simulink model "iasted_s1"  (R2014a)
settings: Solver=ode3  StartTime=0.0  StopTime=10  FixedStep=T  RelTol=1e-3
values from neighbouring files (symbols this model uses):
  amplitude = 10    [iasted_m1.m]
  duracao = 0.1    [iasted_m1.m]
  G = [solution.k1  solution.k2  0  solution.k4]    [iasted_m1.m]
  theta_r = 1.0    (= 1)    [iasted_m1.m]
  ti = 10    [iasted_m1.m]
settings Model: Creator=fabrizio  LastModifiedBy=fabrizio
settings DataIOCC: Refine=10

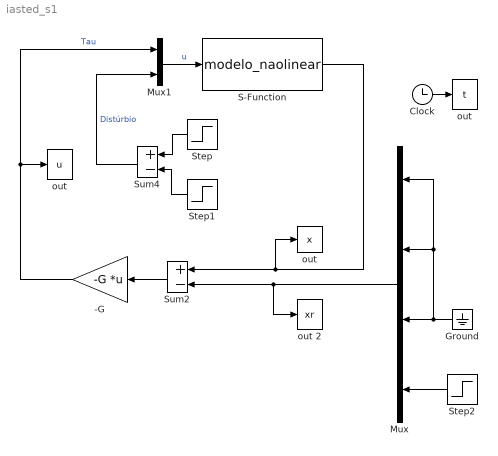
== system iasted_s1 ==
  -G : Gain  Gain=-G  Multiplication=Matrix(K*u)
  Clock : Clock
  Ground : Ground
  Mux : Mux
  Mux1 : Mux  Inputs=2
  S-Function : S-Function  FunctionName=modelo_naolinear  Parameters=pars  EnableBusSupport=off
  Step : Step  Time=ti  After=amplitude  SampleTime=0
  Step1 : Step  Time=ti+duracao  After=amplitude  SampleTime=0
  Step2 : Step  Time=5  After=theta_r  SampleTime=0
  Sum2 : Sum  Inputs=+-
  Sum4 : Sum  Inputs=+-
  out : ToWorkspace  VariableName=t  SampleTime=-1
  "out " : ToWorkspace  VariableName=x  SampleTime=-1
  "out  " : ToWorkspace  VariableName=u  SampleTime=-1
  out 2 : ToWorkspace  VariableName=xr  SampleTime=-1
  wires:
  Sum2/1 -> -G/1
  Clock/1 -> out/1
  Mux/1 -> out 2/1, Sum2/2
  -G/1 -> Mux1/1, "out  "/1  "Tau"
  Step2/1 -> Mux/4
  Mux1/1 -> S-Function/1  "u"
  Step/1 -> Sum4/1
  Step1/1 -> Sum4/2
  S-Function/1 -> "out "/1, Sum2/1
  Ground/1 -> Mux/3, Mux/1, Mux/2
  Sum4/1 -> Mux1/2  "Distúrbio"
